simulink model "lab07es02_schema"  (R2021b)
settings: Solver=VariableStepAuto  StartTime=0.0  StopTime=50  RelTol=1e-3
values from neighbouring files (symbols this model uses):
  Kr = 1    [L_11_05_21_reti_anticipatrici.m]    (also in L_11_05_21_reti_anticipatrici_2.m; L_12_05_21_Esercizio_progetto_di_un_controllore.m; L_12_05_21_effetti_sul_comando.m; L_12_05_21_reti_integro-derivative.m)
libraries: cstblocks x2, simulink x1
settings Model: Creator=armandofornasier  LastModifiedBy=francescafornasier

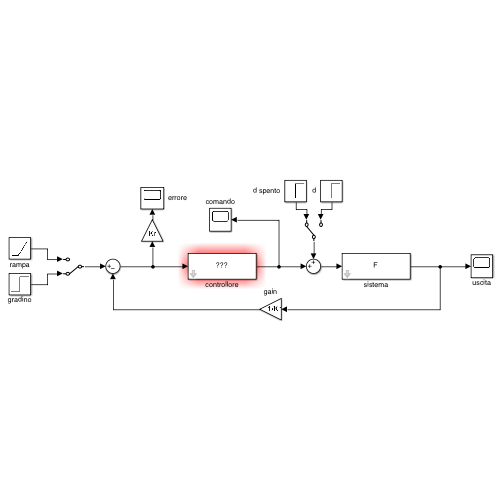
[thumbnail: Simulink's stored preview of the top-level diagram]
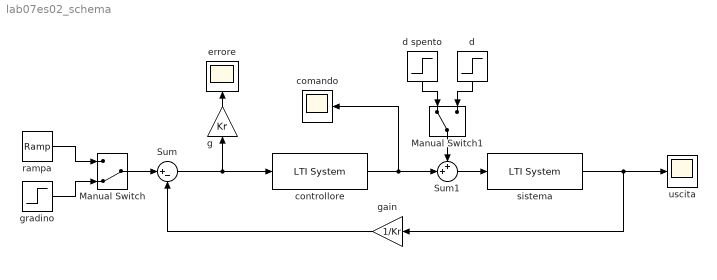
== system lab07es02_schema ==
  Manual Switch : ManualSwitch  CurrentSetting=0
  Manual Switch1 : ManualSwitch
  Sum : Sum  Inputs=|+-
  Sum1 : Sum  Inputs=++|
  comando : Scope
  controllore : cstblocks/LTI System  sys=C  IC=[]
  d : Step  Time=0  SampleTime=0
  d spento : Step  Time=0  After=0  SampleTime=0
  errore : Scope
  g : Gain  Gain=Kr
  gain : Gain  Gain=1/Kr
  gradino : Step  Time=0  SampleTime=0
  rampa : simulink/Sources/Ramp  slope=1  start=0  InitialOutput=0
  sistema : cstblocks/LTI System  sys=F  IC=[]
  uscita : Scope
  wires:
  Sum/1 -> g/1, controllore/1
  gain/1 -> Sum/2
  Sum1/1 -> sistema/1
  sistema/1 -> uscita/1, gain/1
  Manual Switch/1 -> Sum/1
  rampa/1 -> Manual Switch/1
  gradino/1 -> Manual Switch/2
  Manual Switch1/1 -> Sum1/1
  d/1 -> Manual Switch1/2
  d spento/1 -> Manual Switch1/1
  g/1 -> errore/1
  controllore/1 -> comando/1, Sum1/2
